simulink model "MultipleSourcesTransition"  (R2020b)
settings: Solver=VariableStepAuto  StartTime=0.0  StopTime=10.0  RelTol=1e-3
settings Model: Creator=apple  LastModifiedBy=apple

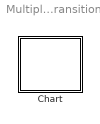
== system MultipleSourcesTransition ==
  Chart : Stateflow chart  TreatAsAtomicUnit=on

== stateflow chart MultipleSourcesTransition/Chart ==
  state A
    en:fprintf("Entry A");
    du:fprintf("During A");
    ex:fprintf("Exit A");
  state C
    en:fprintf("Entry C");
    du:fprintf("During C");
    ex:fprintf("Exit A");
  state B
    en:fprintf("Entry B");
    du:fprintf("During B");
    ex:fprintf("Exit B");
  (default) -> A
  A -> (junction 6) : E_one
  (junction 6) -> C
  B -> (junction 6) : E_two
  events: E_one local FUNCTION_CALL_EVENT; E_two local FUNCTION_CALL_EVENT
